simulink library "str"  (Simulink 8.2)
settings: Solver=ode45  SolverMode=SingleTasking  StartTime=0.0  StopTime=10.0  RelTol=1e-3
undefined symbols (not defined in the file or in its folder): ASTR_LFCTransGainIPTq_X_Nm, ASTR_LFCTransGainOPTq_X_Nm, ENUM_ADASLFCSTATUS_ACTIVE_NORMAL, ENUM_EPSMODEREQ_TORQUE, ENUM_LFCSTATE_SOFTEN, FALSE, KINP_SteerSpeedCalRate_s, KINP_SteerSpeedFltConst_s, KSTR_AngSvoErrGain_rat, KSTR_AngSvoFFVal_degps, KSTR_AngSvoIC_degps, KSTR_AngSvoIGain_rat, KSTR_AngSvoIMax_degps, KSTR_AngSvoIMin_degps, KSTR_AngSvoKGain_rat, KSTR_AngSvoPGain_rat, KSTR_ForceAngleServoOn_flg, KSTR_StrAngComdGain_rat, KSTR_StrAngGain_rat, KSTR_StrSpdGain_rat, KSTR_UseFakeStrAngReq_flg, MSTR_LFCTransGainIP_rat, MSTR_LFCTransGainOP_rat, TRUE
libraries: hcu_lib x6, simulink x3, inp x1
settings Model: Creator=13192  LastModifiedBy=13192

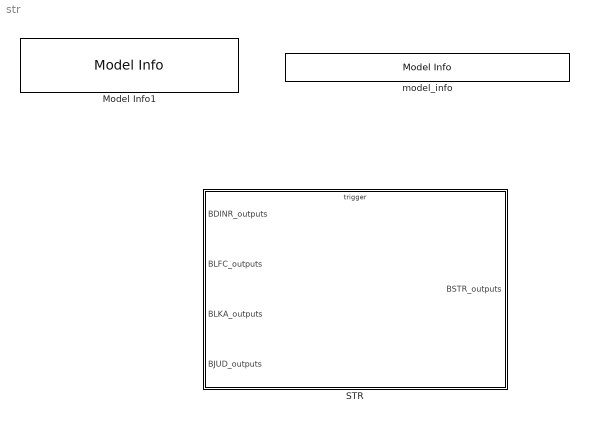
== system str ==
  Model Info1 : simulink/Model-Wide Utilities/Model Info  InitialBlockCM=None  BlockCM=None  Frame=on  DisplayStringWithTags=|  HorizontalTextAlignment=Left  LeftAlignmentValue=0.02  SourceBlockDiagram=str  TagMaxNumber=20
      | Model Version        : %<ModelVersion>
      | Creator                   : %<Creator>
      | Last Modified by    : %<LastModifiedBy>
  STR : Subsystem
      settings: RTWSystemCode=Nonreusable function  RTWFcnNameOpts=Use subsystem name  RTWFileNameOpts=Use subsystem name
  model_info : simulink/Model-Wide Utilities/Model Info  InitialBlockCM=None  BlockCM=None  Frame=on  DisplayStringWithTags=$Id: hcu_lib.mdl 289 2016-04-11 06:01:08Z chimotsai $  HorizontalTextAlignment=Center  LeftAlignmentValue=0.5  SourceBlockDiagram=str  TagMaxNumber=20

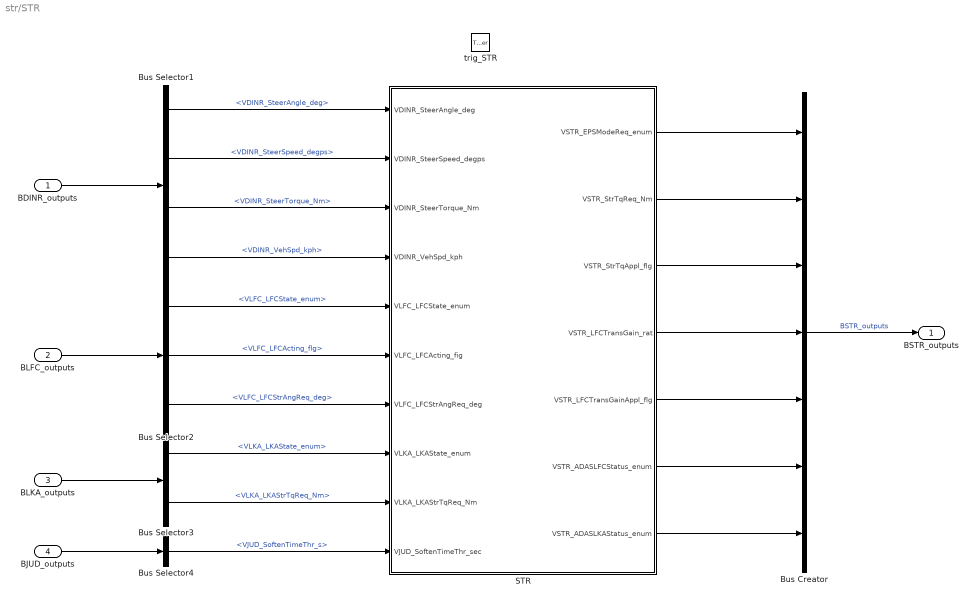
== system str/STR ==
  BDINR_outputs : Inport  OutDataTypeStr=Bus: BDINR_outputs
  BLFC_outputs : Inport  Port=2  OutDataTypeStr=Bus: BLFC_outputs
  BLKA_outputs : Inport  Port=3  OutDataTypeStr=Bus: BLKA_outputs
  BJUD_outputs : Inport  Port=4  OutDataTypeStr=Bus: BJUD_outputs
  trig_STR : TriggerPort  TriggerType=function-call
  Bus Creator : BusCreator  Inputs=7  OutDataTypeStr=Bus: BSTR_outputs
  Bus Selector1 : BusSelector  OutputSignals=VDINR_SteerAngle_deg,VDINR_SteerSpeed_degps,VDINR_SteerTorque_Nm,VDINR_VehSpd_kph
  Bus Selector2 : BusSelector  OutputSignals=VLFC_LFCState_enum,VLFC_LFCActing_flg,VLFC_LFCStrAngReq_deg
  Bus Selector3 : BusSelector  OutputSignals=VLKA_LKAState_enum,VLKA_LKAStrTqReq_Nm
  Bus Selector4 : BusSelector  OutputSignals=VJUD_SoftenTimeThr_s
  STR : Subsystem
  BSTR_outputs : Outport  OutDataTypeStr=Bus: BSTR_outputs
  wires:
  Bus Creator/1 -> BSTR_outputs/1  "BSTR_outputs"
  BDINR_outputs/1 -> Bus Selector1/1
  Bus Selector1/1 -> STR/1(VDINR_SteerAngle_deg)  "<VDINR_SteerAngle_deg>"
  Bus Selector1/2 -> STR/2(VDINR_SteerSpeed_degps)  "<VDINR_SteerSpeed_degps>"
  BLFC_outputs/1 -> Bus Selector2/1
  Bus Selector1/4 -> STR/4(VDINR_VehSpd_kph)  "<VDINR_VehSpd_kph>"
  Bus Selector2/1 -> STR/5(VLFC_LFCState_enum)  "<VLFC_LFCState_enum>"
  Bus Selector2/3 -> STR/7(VLFC_LFCStrAngReq_deg)  "<VLFC_LFCStrAngReq_deg>"
  BLKA_outputs/1 -> Bus Selector3/1
  Bus Selector3/1 -> STR/8(VLKA_LKAState_enum)  "<VLKA_LKAState_enum>"
  Bus Selector3/2 -> STR/9(VLKA_LKAStrTqReq_Nm)  "<VLKA_LKAStrTqReq_Nm>"
  Bus Selector1/3 -> STR/3(VDINR_SteerTorque_Nm)  "<VDINR_SteerTorque_Nm>"
  BJUD_outputs/1 -> Bus Selector4/1
  Bus Selector4/1 -> STR/10(VJUD_SoftenTimeThr_sec)  "<VJUD_SoftenTimeThr_s>"
  STR/1(VSTR_EPSModeReq_enum) -> Bus Creator/1
  STR/2(VSTR_StrTqReq_Nm) -> Bus Creator/2
  STR/3(VSTR_StrTqAppl_flg) -> Bus Creator/3
  STR/4(VSTR_LFCTransGain_rat) -> Bus Creator/4
  STR/5(VSTR_LFCTransGainAppl_flg) -> Bus Creator/5
  STR/6(VSTR_ADASLFCStatus_enum) -> Bus Creator/6
  STR/7(VSTR_ADASLKAStatus_enum) -> Bus Creator/7
  Bus Selector2/2 -> STR/6(VLFC_LFCActing_fig)  "<VLFC_LFCActing_flg>"

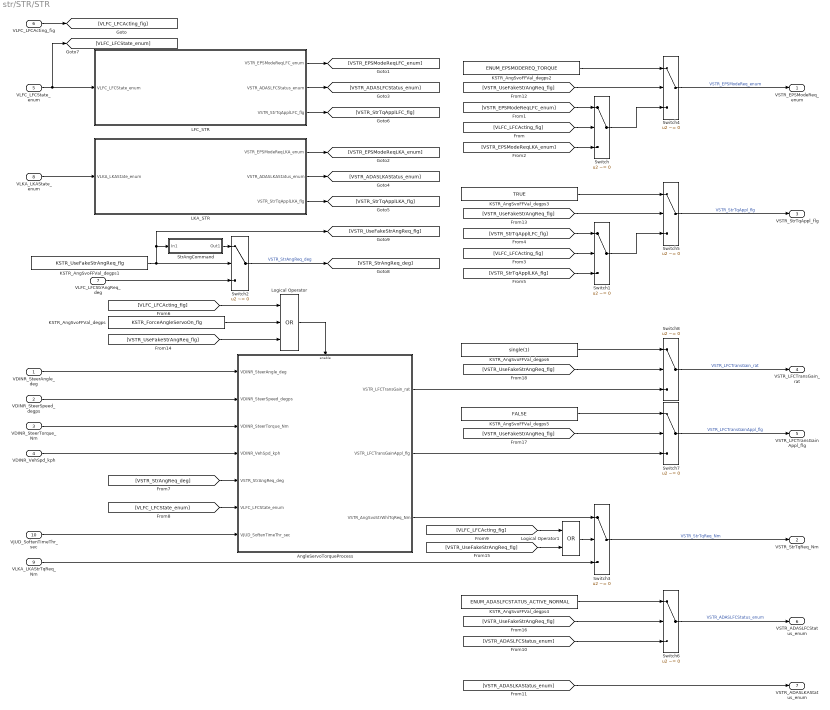
== system str/STR/STR ==
  VDINR_SteerAngle_deg : Inport
  VDINR_SteerSpeed_degps : Inport  Port=2
  VDINR_SteerTorque_Nm : Inport  Port=3
  VDINR_VehSpd_kph : Inport  Port=4
  VLFC_LFCState_enum : Inport  Port=5
  VLFC_LFCActing_fig : Inport  Port=6
  VLFC_LFCStrAngReq_deg : Inport  Port=7
  VLKA_LKAState_enum : Inport  Port=8
  VLKA_LKAStrTqReq_Nm : Inport  Port=9
  VJUD_SoftenTimeThr_sec : Inport  Port=10
  AngleServoTorqueProcess : Subsystem
  KSTR_AngSvoFFVal_degps : Constant  Value=KSTR_ForceAngleServoOn_flg
  KSTR_AngSvoFFVal_degps1 : Constant  Value=KSTR_UseFakeStrAngReq_flg
  KSTR_AngSvoFFVal_degps2 : Constant  Value=ENUM_EPSMODEREQ_TORQUE
  KSTR_AngSvoFFVal_degps3 : Constant  Value=TRUE
  KSTR_AngSvoFFVal_degps4 : Constant  Value=ENUM_ADASLFCSTATUS_ACTIVE_NORMAL
  KSTR_AngSvoFFVal_degps5 : Constant  Value=FALSE
  KSTR_AngSvoFFVal_degps6 : Constant  Value=single(1)
  LFC_STR : Stateflow chart  TreatAsAtomicUnit=on
  LKA_STR : Stateflow chart  TreatAsAtomicUnit=on
  Logical Operator : Logic  Operator=OR  Inputs=3  AllPortsSameDT=off  OutDataTypeStr=boolean
  Logical Operator1 : Logic  Operator=OR  AllPortsSameDT=off  OutDataTypeStr=boolean
  StrAngCommand : Subsystem
  Switch{,1..8} (9 alike) : Switch  Criteria=u2 ~= 0
  VSTR_EPSModeReq_enum : Outport
  VSTR_StrTqReq_Nm : Outport  Port=2
  VSTR_StrTqAppl_flg : Outport  Port=3
  VSTR_LFCTransGain_rat : Outport  Port=4
  VSTR_LFCTransGainAppl_flg : Outport  Port=5
  VSTR_ADASLFCStatus_enum : Outport  Port=6
  VSTR_ADASLKAStatus_enum : Outport  Port=7
  wires:
  VLKA_LKAState_enum/1 -> LKA_STR/1(VLKA_LKAState_enum)
  VLFC_LFCState_enum/1 -> [VLFC_LFCState_enum], LFC_STR/1(VLFC_LFCState_enum)
  VLFC_LFCActing_fig/1 -> [VLFC_LFCActing_fig]
  LFC_STR/1(VSTR_EPSModeReqLFC_enum) -> [VSTR_EPSModeReqLFC_enum]
  LKA_STR/1(VSTR_EPSModeReqLKA_enum) -> [VSTR_EPSModeReqLKA_enum]
  LFC_STR/2(VSTR_ADASLFCStatus_enum) -> [VSTR_ADASLFCStatus_enum]
  LKA_STR/2(VSTR_ADASLKAStatus_enum) -> [VSTR_ADASLKAStatus_enum]
  LKA_STR/3(VSTR_StrTqApplLKA_flg) -> [VSTR_StrTqApplLKA_flg]
  LFC_STR/3(VSTR_StrTqApplLFC_flg) -> [VSTR_StrTqApplLFC_flg]
  [VLFC_LFCActing_fig] -> Switch/2
  [VSTR_EPSModeReqLFC_enum] -> Switch/1
  [VSTR_EPSModeReqLKA_enum] -> Switch/3
  [VLFC_LFCActing_fig] -> Switch1/2
  [VSTR_StrTqApplLFC_flg] -> Switch1/1
  [VSTR_StrTqApplLKA_flg] -> Switch1/3
  Switch4/1 -> VSTR_EPSModeReq_enum/1  "VSTR_EPSModeReq_enum"
  Switch5/1 -> VSTR_StrTqAppl_flg/1  "VSTR_StrTqAppl_flg"
  Logical Operator/1 -> AngleServoTorqueProcess/Enable
  [VLFC_LFCActing_fig] -> Logical Operator/1
  KSTR_AngSvoFFVal_degps/1 -> Logical Operator/2
  VDINR_SteerAngle_deg/1 -> AngleServoTorqueProcess/1(VDINR_SteerAngle_deg)
  VDINR_SteerSpeed_degps/1 -> AngleServoTorqueProcess/2(VDINR_SteerSpeed_degps)
  VDINR_SteerTorque_Nm/1 -> AngleServoTorqueProcess/3(VDINR_SteerTorque_Nm)
  VDINR_VehSpd_kph/1 -> AngleServoTorqueProcess/4(VDINR_VehSpd_kph)
  KSTR_AngSvoFFVal_degps1/1 -> StrAngCommand/1(In1), [VSTR_UseFakeStrAngReq_flg], Switch2/2
  StrAngCommand/1(Out1) -> Switch2/1
  Switch2/1 -> [VSTR_StrAngReq_deg]  "VSTR_StrAngReq_deg"
  [VSTR_StrAngReq_deg] -> AngleServoTorqueProcess/5(VSTR_StrAngReq_deg)
  [VLFC_LFCState_enum] -> AngleServoTorqueProcess/6(VLFC_LFCState_enum)
  VJUD_SoftenTimeThr_sec/1 -> AngleServoTorqueProcess/7(VJUD_SoftenTimeThr_sec)
  VLKA_LKAStrTqReq_Nm/1 -> Switch3/3
  AngleServoTorqueProcess/3(VSTR_AngSvoStrWhlTqReq_Nm) -> Switch3/1
  Switch3/1 -> VSTR_StrTqReq_Nm/1  "VSTR_StrTqReq_Nm"
  AngleServoTorqueProcess/1(VSTR_LFCTransGain_rat) -> Switch8/3
  AngleServoTorqueProcess/2(VSTR_LFCTransGainAppl_flg) -> Switch7/3
  [VSTR_ADASLFCStatus_enum] -> Switch6/3
  [VSTR_ADASLKAStatus_enum] -> VSTR_ADASLKAStatus_enum/1
  [VSTR_UseFakeStrAngReq_flg] -> Switch4/2
  Switch/1 -> Switch4/3
  KSTR_AngSvoFFVal_degps2/1 -> Switch4/1
  [VSTR_UseFakeStrAngReq_flg] -> Switch5/2
  Switch1/1 -> Switch5/3
  KSTR_AngSvoFFVal_degps3/1 -> Switch5/1
  [VSTR_UseFakeStrAngReq_flg] -> Logical Operator/3
  Logical Operator1/1 -> Switch3/2
  [VLFC_LFCActing_fig] -> Logical Operator1/1
  [VSTR_UseFakeStrAngReq_flg] -> Logical Operator1/2
  [VSTR_UseFakeStrAngReq_flg] -> Switch6/2
  KSTR_AngSvoFFVal_degps4/1 -> Switch6/1
  Switch6/1 -> VSTR_ADASLFCStatus_enum/1  "VSTR_ADASLFCStatus_enum"
  [VSTR_UseFakeStrAngReq_flg] -> Switch7/2
  KSTR_AngSvoFFVal_degps5/1 -> Switch7/1
  Switch7/1 -> VSTR_LFCTransGainAppl_flg/1  "VSTR_LFCTransGainAppl_flg"
  [VSTR_UseFakeStrAngReq_flg] -> Switch8/2
  KSTR_AngSvoFFVal_degps6/1 -> Switch8/1
  Switch8/1 -> VSTR_LFCTransGain_rat/1  "VSTR_LFCTransGain_rat"
  VLFC_LFCStrAngReq_deg/1 -> Switch2/3

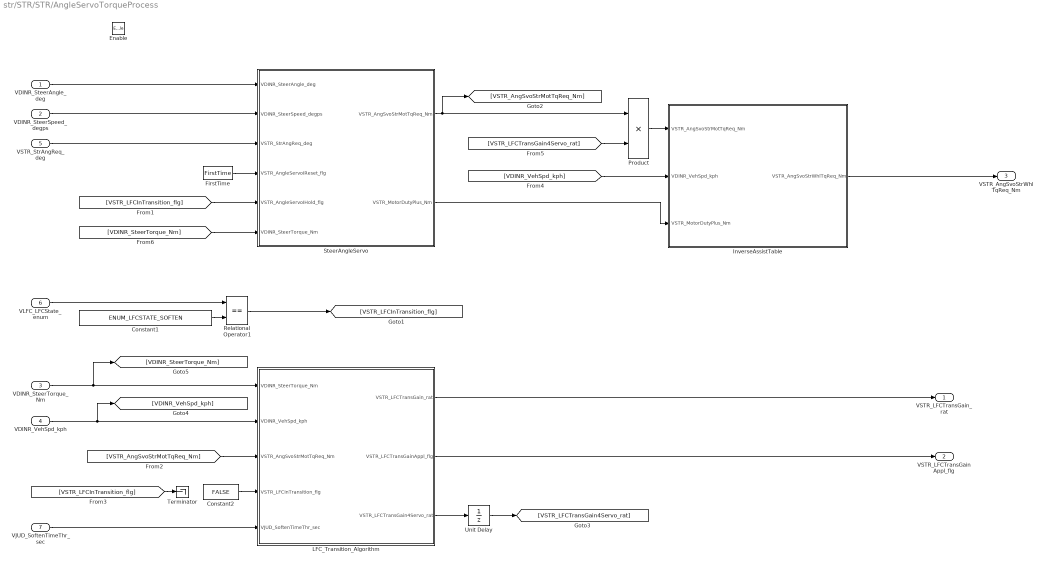
== system str/STR/STR/AngleServoTorqueProcess ==
  VDINR_SteerAngle_deg : Inport
  VDINR_SteerSpeed_degps : Inport  Port=2
  VDINR_SteerTorque_Nm : Inport  Port=3
  VDINR_VehSpd_kph : Inport  Port=4
  VSTR_StrAngReq_deg : Inport  Port=5
  VLFC_LFCState_enum : Inport  Port=6
  VJUD_SoftenTimeThr_sec : Inport  Port=7
  Enable : EnablePort  StatesWhenEnabling=reset
  Constant1 : Constant  Value=ENUM_LFCSTATE_SOFTEN
  Constant2 : Constant  Value=FALSE
  FirstTime : hcu_lib/FirstTime
  InverseAssistTable : Subsystem
  LFC_Transition_Algorithm : Subsystem
  Product : Product  Inputs=**
  Relational Operator1 : RelationalOperator  Operator===  OutDataTypeStr=boolean
  SteerAngleServo : Subsystem
  Terminator : Terminator
  Unit Delay : UnitDelay  InitialCondition=1  SampleTime=-1
  VSTR_LFCTransGain_rat : Outport  OutputWhenDisabled=reset  InitialOutput=[1]
  VSTR_LFCTransGainAppl_flg : Outport  Port=2  OutputWhenDisabled=reset  InitialOutput=[0]
  VSTR_AngSvoStrWhlTqReq_Nm : Outport  Port=3  OutputWhenDisabled=reset  InitialOutput=[0]
  wires:
  SteerAngleServo/1(VSTR_AngSvoStrMotTqReq_Nm) -> [VSTR_AngSvoStrMotTqReq_Nm], Product/1
  VDINR_SteerSpeed_degps/1 -> SteerAngleServo/2(VDINR_SteerSpeed_degps)
  VSTR_StrAngReq_deg/1 -> SteerAngleServo/3(VSTR_StrAngReq_deg)
  VDINR_SteerAngle_deg/1 -> SteerAngleServo/1(VDINR_SteerAngle_deg)
  InverseAssistTable/1(VSTR_AngSvoStrWhlTqReq_Nm) -> VSTR_AngSvoStrWhlTqReq_Nm/1
  FirstTime/1 -> SteerAngleServo/4(VSTR_AngleServoIReset_flg)
  VLFC_LFCState_enum/1 -> Relational Operator1/1
  Constant1/1 -> Relational Operator1/2
  [VSTR_LFCInTransition_flg] -> SteerAngleServo/5(VSTR_AngleServoIHold_flg)
  VDINR_VehSpd_kph/1 -> [VDINR_VehSpd_kph], LFC_Transition_Algorithm/2(VDINR_VehSpd_kph)
  VDINR_SteerTorque_Nm/1 -> [VDINR_SteerTorque_Nm], LFC_Transition_Algorithm/1(VDINR_SteerTorque_Nm)
  [VSTR_AngSvoStrMotTqReq_Nm] -> LFC_Transition_Algorithm/3(VSTR_AngSvoStrMotTqReq_Nm)
  [VSTR_LFCInTransition_flg] -> Terminator/1
  VJUD_SoftenTimeThr_sec/1 -> LFC_Transition_Algorithm/5(VJUD_SoftenTimeThr_sec)
  LFC_Transition_Algorithm/3(VSTR_LFCTransGain4Servo_rat) -> Unit Delay/1
  LFC_Transition_Algorithm/1(VSTR_LFCTransGain_rat) -> VSTR_LFCTransGain_rat/1
  LFC_Transition_Algorithm/2(VSTR_LFCTransGainAppl_flg) -> VSTR_LFCTransGainAppl_flg/1
  Unit Delay/1 -> [VSTR_LFCTransGain4Servo_rat]
  [VDINR_VehSpd_kph] -> InverseAssistTable/2(VDINR_VehSpd_kph)
  Product/1 -> InverseAssistTable/1(VSTR_AngSvoStrMotTqReq_Nm)
  [VSTR_LFCTransGain4Servo_rat] -> Product/2
  Constant2/1 -> LFC_Transition_Algorithm/4(VSTR_LFCInTransition_flg)
  SteerAngleServo/2(VSTR_MotorDutyPlus_Nm) -> InverseAssistTable/3(VSTR_MotorDutyPlus_Nm)
  Relational Operator1/1 -> [VSTR_LFCInTransition_flg]
  [VDINR_SteerTorque_Nm] -> SteerAngleServo/6(VDINR_SteerTorque_Nm)

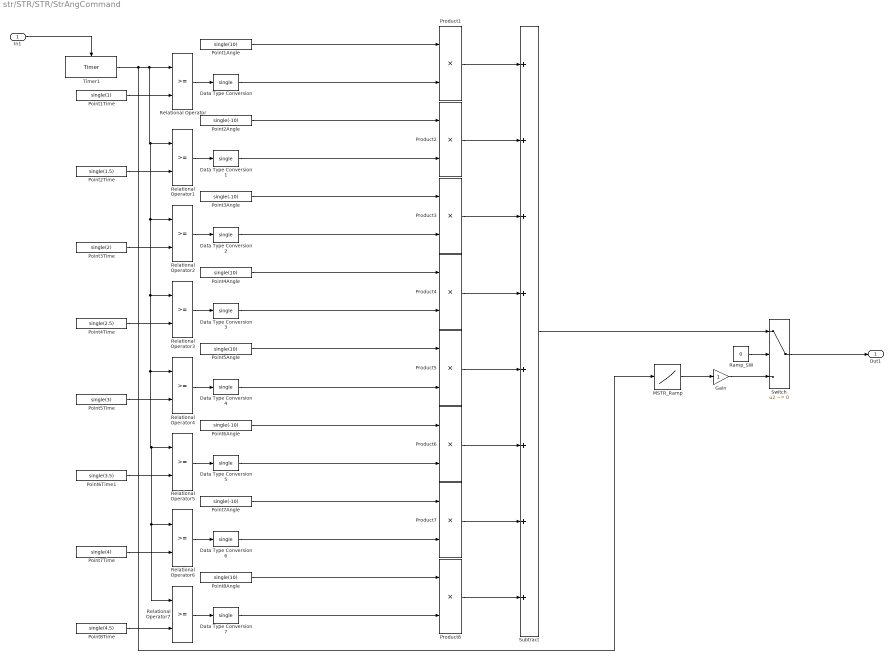
== system str/STR/STR/StrAngCommand ==
  In1 : Inport
  Data Type Conversion{,1..7} (8 alike) : DataTypeConversion  OutDataTypeStr=single
  Gain : Gain
  MSTR_Ramp : Lookup  InputValues=[0.5 1 1.1 3]  Table=[0 0 1 1]  LookUpMeth=Interpolation-Use End Values
      settings: AttributesFormatString="Input=\"%<InputValues>\"\\nOutput=\"%<Table>\""
  Point1Angle : Constant  Value=single(10)
  Point1Time : Constant  Value=single(1)
  Point2Angle : Constant  Value=single(-10)
  Point2Time : Constant  Value=single(1.5)
  Point3Angle : Constant  Value=single(-10)
  Point3Time : Constant  Value=single(2)
  Point4Angle : Constant  Value=single(10)
  Point4Time : Constant  Value=single(2.5)
  Point5Angle : Constant  Value=single(10)
  Point5Time : Constant  Value=single(3)
  Point6Angle : Constant  Value=single(-10)
  Point6Time1 : Constant  Value=single(3.5)
  Point7Angle : Constant  Value=single(-10)
  Point7Time : Constant  Value=single(4)
  Point8Angle : Constant  Value=single(10)
  Point8Time : Constant  Value=single(4.5)
  Product{1..8} (8 alike) : Product
  Ramp_SW : Constant  Value=0  OutDataTypeStr=boolean
  Relational Operator{,1..7} (8 alike) : RelationalOperator  OutDataTypeStr=boolean
  Subtract : Sum  Inputs=8
  Switch : Switch  Criteria=u2 ~= 0
  Timer1 : hcu_lib/Timer  SystemSampleTime=-1
  Out1 : Outport
  wires:
  In1/1 -> Timer1/Enable
  Point1Time/1 -> Relational Operator/2
  Relational Operator/1 -> Data Type Conversion/1
  Data Type Conversion/1 -> Product1/2
  Point1Angle/1 -> Product1/1
  Point2Time/1 -> Relational Operator1/2
  Data Type Conversion1/1 -> Product2/2
  Point2Angle/1 -> Product2/1
  Relational Operator1/1 -> Data Type Conversion1/1
  Point3Time/1 -> Relational Operator2/2
  Data Type Conversion2/1 -> Product3/2
  Relational Operator2/1 -> Data Type Conversion2/1
  Point3Angle/1 -> Product3/1
  Point4Time/1 -> Relational Operator3/2
  Data Type Conversion3/1 -> Product4/2
  Relational Operator3/1 -> Data Type Conversion3/1
  Point4Angle/1 -> Product4/1
  Point5Time/1 -> Relational Operator4/2
  Data Type Conversion4/1 -> Product5/2
  Relational Operator4/1 -> Data Type Conversion4/1
  Point5Angle/1 -> Product5/1
  Point6Time1/1 -> Relational Operator5/2
  Data Type Conversion5/1 -> Product6/2
  Relational Operator5/1 -> Data Type Conversion5/1
  Point6Angle/1 -> Product6/1
  Point7Time/1 -> Relational Operator6/2
  Data Type Conversion6/1 -> Product7/2
  Relational Operator6/1 -> Data Type Conversion6/1
  Point7Angle/1 -> Product7/1
  Timer1/1 -> MSTR_Ramp/1, Relational Operator7/1, Relational Operator6/1, Relational Operator5/1, Relational Operator4/1, Relational Operator3/1, Relational Operator2/1, Relational Operator1/1, Relational Operator/1
  Point8Time/1 -> Relational Operator7/2
  Data Type Conversion7/1 -> Product8/2
  Relational Operator7/1 -> Data Type Conversion7/1
  Point8Angle/1 -> Product8/1
  Product1/1 -> Subtract/1
  Product2/1 -> Subtract/2
  Product3/1 -> Subtract/3
  Product4/1 -> Subtract/4
  Product5/1 -> Subtract/5
  Product6/1 -> Subtract/6
  Product7/1 -> Subtract/7
  Product8/1 -> Subtract/8
  Switch/1 -> Out1/1
  MSTR_Ramp/1 -> Gain/1
  Subtract/1 -> Switch/1
  Gain/1 -> Switch/3
  Ramp_SW/1 -> Switch/2

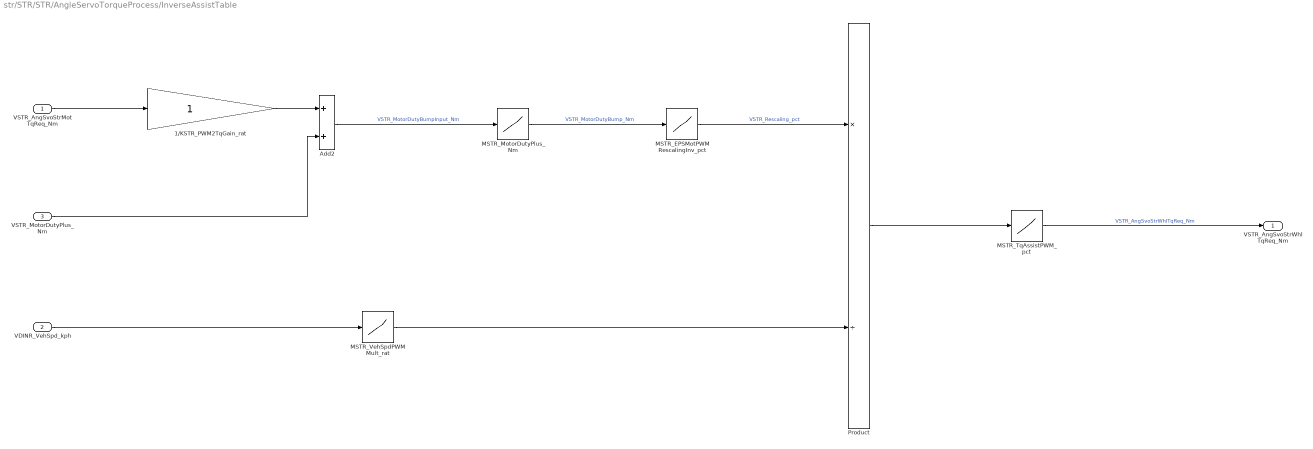
== system str/STR/STR/AngleServoTorqueProcess/InverseAssistTable ==
  VSTR_AngSvoStrMotTqReq_Nm : Inport
  VDINR_VehSpd_kph : Inport  Port=2
  VSTR_MotorDutyPlus_Nm : Inport  Port=3
  1/KSTR_PWM2TqGain_rat : Gain
  Add2 : Sum
  MSTR_EPSMotPWMRescalingInv_pct : Lookup  InputValues=[-250 -3 0 3 250]  Table=[-100 -3 0 3 100]  LookUpMeth=Interpolation-Use End Values
      settings: AttributesFormatString="Input=\"%<InputValues>\"\\nOutput=\"%<Table>\""
  MSTR_MotorDutyPlus_Nm : Lookup  InputValues=[-100 -50 -10 -5 -1 0 1 5 10 50 100]  Table=[-104 -54 -14 -9 -5 0 5 9 14 54 104]  LookUpMeth=Interpolation-Use End Values
      settings: AttributesFormatString="Input=\"%<InputValues>\"\\nOutput=\"%<Table>\""
  MSTR_TqAssistPWM_pct : Lookup  InputValues="[-100\t-95\t-90\t-85\t-80\t-75\t-70\t-65\t-60\t-55\t-50\t-45\t-40\t-35\t-30\t-25\t-20\t-15\t-10\t-5\t0\t5\t10\t15\t20\t25\t30\t35\t40\t45\t50\t55\t60\t65\t70\t75\t80\t85\t90\t95\t100]"  Table=[-10:0.5:10]  LookUpMeth=Interpolation-Use End Values
      settings: AttributesFormatString="Input=\"%<InputValues>\"\\nOutput=\"%<Table>\""
  MSTR_VehSpdPWMMult_rat : Lookup  InputValues=[-100 -80 -60 -40 -20 -10 0 10 20 40 60 80 100]  Table=[1 1 1 1 1 1 1 1 1 1 1 1 1]  LookUpMeth=Interpolation-Use End Values
      settings: AttributesFormatString="Input=\"%<InputValues>\"\\nOutput=\"%<Table>\""
  Product : Product  Inputs=*/
  VSTR_AngSvoStrWhlTqReq_Nm : Outport
  wires:
  VSTR_AngSvoStrMotTqReq_Nm/1 -> 1/KSTR_PWM2TqGain_rat/1
  1/KSTR_PWM2TqGain_rat/1 -> Add2/1
  VDINR_VehSpd_kph/1 -> MSTR_VehSpdPWMMult_rat/1
  MSTR_VehSpdPWMMult_rat/1 -> Product/2
  Product/1 -> MSTR_TqAssistPWM_pct/1
  MSTR_TqAssistPWM_pct/1 -> VSTR_AngSvoStrWhlTqReq_Nm/1  "VSTR_AngSvoStrWhlTqReq_Nm"
  MSTR_EPSMotPWMRescalingInv_pct/1 -> Product/1  "VSTR_Rescaling_pct"
  MSTR_MotorDutyPlus_Nm/1 -> MSTR_EPSMotPWMRescalingInv_pct/1  "VSTR_MotorDutyBump_Nm"
  Add2/1 -> MSTR_MotorDutyPlus_Nm/1  "VSTR_MotorDutyBumpInput_Nm"
  VSTR_MotorDutyPlus_Nm/1 -> Add2/2

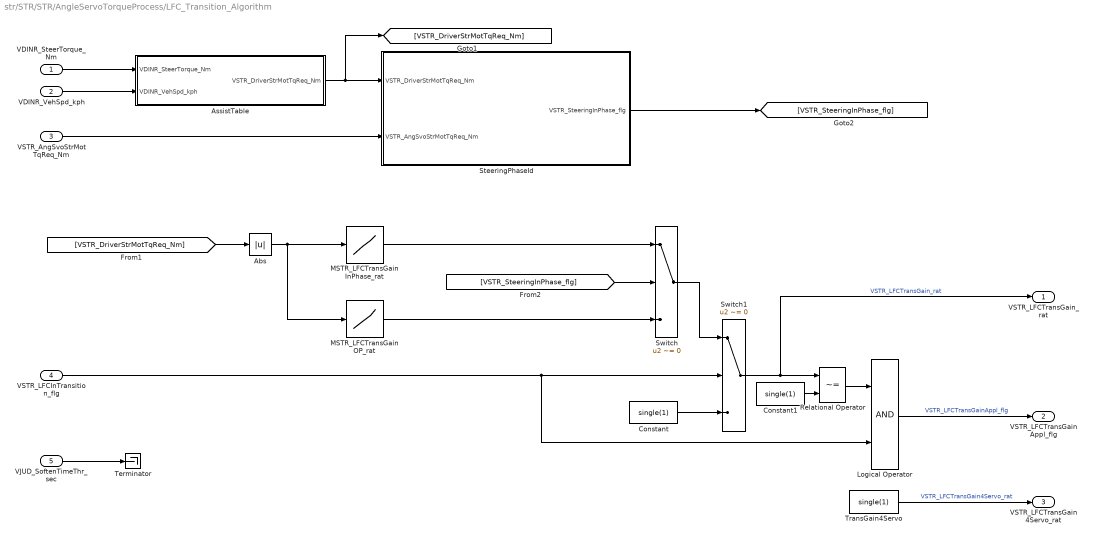
== system str/STR/STR/AngleServoTorqueProcess/LFC_Transition_Algorithm ==
  VDINR_SteerTorque_Nm : Inport
  VDINR_VehSpd_kph : Inport  Port=2
  VSTR_AngSvoStrMotTqReq_Nm : Inport  Port=3
  VSTR_LFCInTransition_flg : Inport  Port=4
  VJUD_SoftenTimeThr_sec : Inport  Port=5
  Abs : Abs
  AssistTable : Subsystem
  Constant : Constant  Value=single(1)
  Constant1 : Constant  Value=single(1)
  Logical Operator : Logic  AllPortsSameDT=off  OutDataTypeStr=boolean
  MSTR_LFCTransGainInPhase_rat : Lookup  InputValues=ASTR_LFCTransGainIPTq_X_Nm  Table=MSTR_LFCTransGainIP_rat  LookUpMeth=Interpolation-Use End Values
      settings: AttributesFormatString="Input=\"%<InputValues>\"\\nOutput=\"%<Table>\""
  MSTR_LFCTransGainOP_rat : Lookup  InputValues=ASTR_LFCTransGainOPTq_X_Nm  Table=MSTR_LFCTransGainOP_rat  LookUpMeth=Interpolation-Use End Values
      settings: AttributesFormatString="Input=\"%<InputValues>\"\\nOutput=\"%<Table>\""
  Relational Operator : RelationalOperator  Operator=~=  OutDataTypeStr=boolean
  SteeringPhaseId : Stateflow chart  TreatAsAtomicUnit=on
  Switch : Switch  Criteria=u2 ~= 0
  Switch1 : Switch  Criteria=u2 ~= 0
  Terminator : Terminator
  TransGain4Servo : Constant  Value=single(1)
  VSTR_LFCTransGain_rat : Outport  OutputWhenDisabled=reset  InitialOutput=[0]
  VSTR_LFCTransGainAppl_flg : Outport  Port=2  OutputWhenDisabled=reset  InitialOutput=[0]
  VSTR_LFCTransGain4Servo_rat : Outport  Port=3  OutputWhenDisabled=reset  InitialOutput=[0]
  wires:
  VSTR_AngSvoStrMotTqReq_Nm/1 -> SteeringPhaseId/2(VSTR_AngSvoStrMotTqReq_Nm)
  VDINR_SteerTorque_Nm/1 -> AssistTable/1(VDINR_SteerTorque_Nm)
  AssistTable/1(VSTR_DriverStrMotTqReq_Nm) -> [VSTR_DriverStrMotTqReq_Nm], SteeringPhaseId/1(VSTR_DriverStrMotTqReq_Nm)
  VDINR_VehSpd_kph/1 -> AssistTable/2(VDINR_VehSpd_kph)
  [VSTR_DriverStrMotTqReq_Nm] -> Abs/1
  Abs/1 -> MSTR_LFCTransGainInPhase_rat/1, MSTR_LFCTransGainOP_rat/1
  SteeringPhaseId/1(VSTR_SteeringInPhase_flg) -> [VSTR_SteeringInPhase_flg]
  [VSTR_SteeringInPhase_flg] -> Switch/2
  MSTR_LFCTransGainInPhase_rat/1 -> Switch/1
  MSTR_LFCTransGainOP_rat/1 -> Switch/3
  VSTR_LFCInTransition_flg/1 -> Logical Operator/2, Switch1/2
  Switch/1 -> Switch1/1
  Constant/1 -> Switch1/3
  Relational Operator/1 -> Logical Operator/1
  Switch1/1 -> VSTR_LFCTransGain_rat/1, Relational Operator/1  "VSTR_LFCTransGain_rat"
  Constant1/1 -> Relational Operator/2
  Logical Operator/1 -> VSTR_LFCTransGainAppl_flg/1  "VSTR_LFCTransGainAppl_flg"
  VJUD_SoftenTimeThr_sec/1 -> Terminator/1
  TransGain4Servo/1 -> VSTR_LFCTransGain4Servo_rat/1  "VSTR_LFCTransGain4Servo_rat"

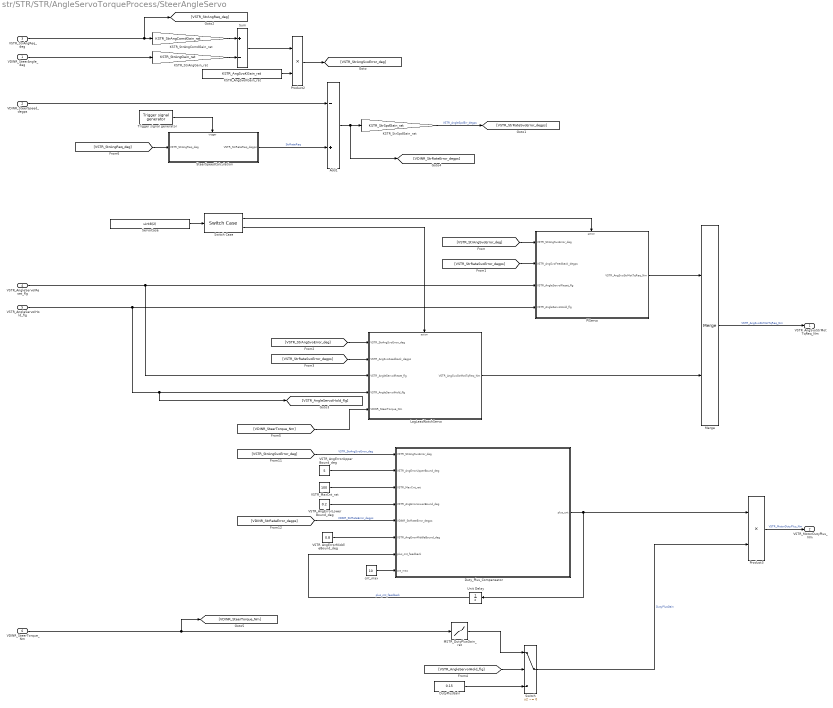
== system str/STR/STR/AngleServoTorqueProcess/SteerAngleServo ==
  VDINR_SteerAngle_deg : Inport
  VDINR_SteerSpeed_degps : Inport  Port=2
  VSTR_StrAngReq_deg : Inport  Port=3
  VSTR_AngleServoIReset_flg : Inport  Port=4
  VSTR_AngleServoIHold_flg : Inport  Port=5
  VDINR_SteerTorque_Nm : Inport  Port=6
  Add1 : Sum  Inputs=-+
  DutyPlusGain : Constant  Value=0.15  OutDataTypeStr=single
  Duty_Plus_Compensator : Stateflow chart  TreatAsAtomicUnit=on
  KSTR_AngSvoKGain_rat : Constant  Value=KSTR_AngSvoKGain_rat
  KSTR_StrAngComdGain_rat : Gain  Gain=KSTR_StrAngComdGain_rat
  KSTR_StrAngGain_rat : Gain  Gain=KSTR_StrAngGain_rat
  KSTR_StrSpdGain_rat : Gain  Gain=KSTR_StrSpdGain_rat
  LagLeadNotchServo : Subsystem
  MSTR_DutyPlusGain_rat : Lookup  InputValues=[1.25 1.5 1.75 2]  Table=[0 0 0 0]  LookUpMeth=Interpolation-Use End Values
      settings: AttributesFormatString="Input=\"%<InputValues>\"\\nOutput=\"%<Table>\""
  Merge : Merge
  PIServo : Subsystem
  Product2 : Product
  Product3 : Product
  ServoCase : Constant  Value=uint8(2)
  SteerSpeedCalculation : Subsystem
  Sum : Sum  Inputs=+-
  Switch : Switch  Criteria=u2 ~= 0
  Switch Case : SwitchCase  CaseConditions={1,2}  ShowDefaultCase=off
  Trigger signal generator : inp/INP/InputSignals/SignalProcess/Proc_SteerSpeedCal/Trigger signal generator
  Unit Delay : UnitDelay  SampleTime=-1
  VSTR_AngErrorLowerBound_deg : Constant  Value=0.2  OutDataTypeStr=single
  VSTR_AngErrorMiddleBound_deg : Constant  Value=0.8  OutDataTypeStr=single
  VSTR_AngErrorUpperBound_deg : Constant  Value=5  OutDataTypeStr=single
  VSTR_MaxCnt_rat : Constant  Value=100  OutDataTypeStr=single
  cnt_max : Constant  Value=10  OutDataTypeStr=single
  VSTR_AngSvoStrMotTqReq_Nm : Outport
  VSTR_MotorDutyPlus_Nm : Outport  Port=2
  wires:
  VSTR_StrAngReq_deg/1 -> [VSTR_StrAngReq_deg], KSTR_StrAngComdGain_rat/1
  KSTR_StrAngComdGain_rat/1 -> Sum/1
  KSTR_StrAngGain_rat/1 -> Sum/2
  Sum/1 -> Product2/1
  KSTR_AngSvoKGain_rat/1 -> Product2/2
  VDINR_SteerAngle_deg/1 -> KSTR_StrAngGain_rat/1
  KSTR_StrSpdGain_rat/1 -> [VSTR_StrRateSvoError_degps]  "VSTR_AngleSpdErr_degps"
  Product2/1 -> [VSTR_StrAngSvoError_deg]
  [VSTR_StrAngSvoError_deg] -> PIServo/1(VSTR_StrAngSvoError_deg)
  [VSTR_StrRateSvoError_degps] -> PIServo/2(VSTR_AngSvoFeedback_degps)
  VSTR_AngleServoIReset_flg/1 -> LagLeadNotchServo/3(VSTR_AngleServoIReset_flg), PIServo/3(VSTR_AngleServoIReset_flg)
  VSTR_AngleServoIHold_flg/1 -> LagLeadNotchServo/4(VSTR_AngleServoIHold_flg), [VSTR_AngleServoIHold_flg], PIServo/4(VSTR_AngleServoIHold_flg)
  PIServo/1(VSTR_AngSvoStrMotTqReq_Nm) -> Merge/1
  [VSTR_StrAngSvoError_deg] -> LagLeadNotchServo/1(VSTR_StrAngSvoError_deg)
  ServoCase/1 -> Switch Case/1
  Merge/1 -> VSTR_AngSvoStrMotTqReq_Nm/1  "VSTR_AngSvoStrMotTqReq_Nm"
  LagLeadNotchServo/1(VSTR_AngSvoStrMotTqReq_Nm) -> Merge/2
  Add1/1 -> KSTR_StrSpdGain_rat/1, [VDINR_StrRateError_degps]
  Trigger signal generator/1 -> SteerSpeedCalculation/Trigger
  [VSTR_StrAngReq_deg] -> SteerSpeedCalculation/1(VSTR_StrAngReq_deg)
  SteerSpeedCalculation/1(VSTR_StrRateReq_degps) -> Add1/2  "StrRateReq"
  [VSTR_StrRateSvoError_degps] -> LagLeadNotchServo/2(VSTR_AngSvoFeedback_degps)
  VDINR_SteerSpeed_degps/1 -> Add1/1
  [VSTR_StrAngSvoError_deg] -> Duty_Plus_Compensator/1(VSTR_StrAngSvoError_deg)  "VSTR_StrAngSvoError_deg"
  Duty_Plus_Compensator/1(plus_cnt) -> Unit Delay/1, Product3/1
  Product3/1 -> VSTR_MotorDutyPlus_Nm/1  "VSTR_MotorDutyPlus_Nm"
  VSTR_AngErrorUpperBound_deg/1 -> Duty_Plus_Compensator/2(VSTR_AngErrorUpperBound_deg)
  VSTR_MaxCnt_rat/1 -> Duty_Plus_Compensator/3(VSTR_MaxCnt_rat)
  VSTR_AngErrorLowerBound_deg/1 -> Duty_Plus_Compensator/4(VSTR_AngErrorLowerBound_deg)
  VSTR_AngErrorMiddleBound_deg/1 -> Duty_Plus_Compensator/6(VSTR_AngErrorMiddleBound_deg)
  [VDINR_StrRateError_degps] -> Duty_Plus_Compensator/5(VDINR_StrRateError_degps)  "VDINR_StrRateError_degps"
  Switch Case/1 -> PIServo/Action
  Switch Case/2 -> LagLeadNotchServo/Action
  Unit Delay/1 -> Duty_Plus_Compensator/7(plus_cnt_feedback)  "plus_cnt_feedback"
  cnt_max/1 -> Duty_Plus_Compensator/8(cnt_max)
  Switch/1 -> Product3/2  "DutyPlusGain"
  DutyPlusGain/1 -> Switch/3
  [VSTR_AngleServoIHold_flg] -> Switch/2
  MSTR_DutyPlusGain_rat/1 -> Switch/1
  VDINR_SteerTorque_Nm/1 -> [VDINR_SteerTorque_Nm], MSTR_DutyPlusGain_rat/1
  [VDINR_SteerTorque_Nm] -> LagLeadNotchServo/5(VDINR_SteerTorque_Nm)

== system str/STR/STR/AngleServoTorqueProcess/LFC_Transition_Algorithm/AssistTable ==
  VDINR_SteerTorque_Nm : Inport
  VDINR_VehSpd_kph : Inport  Port=2
  KSTR_PWM2TqGain_rat : Gain
  MSTR_MotorPWMRescaling_pct : Lookup  InputValues=[-100 -3 0 3 100]  Table=[-250 -3 0 3 250]  LookUpMeth=Interpolation-Use End Values
      settings: AttributesFormatString="Input=\"%<InputValues>\"\\nOutput=\"%<Table>\""
  MSTR_TqPWM_pct : Lookup  InputValues=[-10:0.5:10]  Table="[-100\t-95\t-90\t-85\t-80\t-75\t-70\t-65\t-60\t-55\t-50\t-45\t-40\t-35\t-30\t-25\t-20\t-15\t-10\t-5\t0\t5\t10\t15\t20\t25\t30\t35\t40\t45\t50\t55\t60\t65\t70\t75\t80\t85\t90\t95\t100]"  LookUpMeth=Interpolation-Use End Values
      settings: AttributesFormatString="Input=\"%<InputValues>\"\\nOutput=\"%<Table>\""
  MSTR_VehSpdPWMMult_rat : Lookup  InputValues=[-100 -80 -60 -40 -20 -10 0 10 20 40 60 80 100]  Table=[1 1 1 1 1 1 1 1 1 1 1 1 1]  LookUpMeth=Interpolation-Use End Values
      settings: AttributesFormatString="Input=\"%<InputValues>\"\\nOutput=\"%<Table>\""
  Product : Product  Inputs=**
  VSTR_DriverStrMotTqReq_Nm : Outport
  wires:
  VDINR_VehSpd_kph/1 -> MSTR_VehSpdPWMMult_rat/1
  MSTR_VehSpdPWMMult_rat/1 -> Product/2
  KSTR_PWM2TqGain_rat/1 -> VSTR_DriverStrMotTqReq_Nm/1  "VSTR_DriverStrMotTqReq_Nm"
  VDINR_SteerTorque_Nm/1 -> MSTR_TqPWM_pct/1
  MSTR_TqPWM_pct/1 -> Product/1
  MSTR_MotorPWMRescaling_pct/1 -> KSTR_PWM2TqGain_rat/1
  Product/1 -> MSTR_MotorPWMRescaling_pct/1

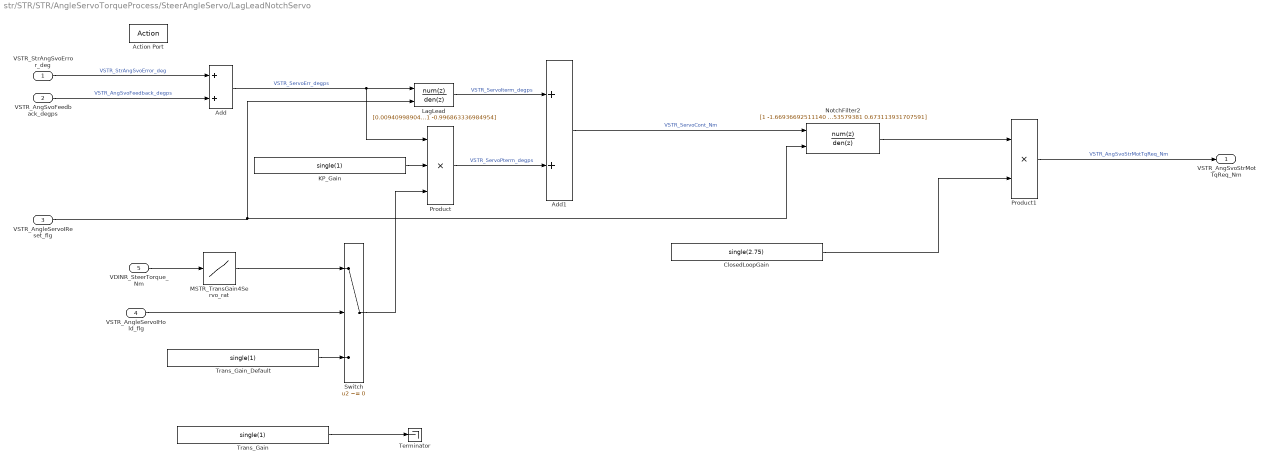
== system str/STR/STR/AngleServoTorqueProcess/SteerAngleServo/LagLeadNotchServo ==
  VSTR_StrAngSvoError_deg : Inport
  VSTR_AngSvoFeedback_degps : Inport  Port=2
  VSTR_AngleServoIReset_flg : Inport  Port=3
  VSTR_AngleServoIHold_flg : Inport  Port=4
  VDINR_SteerTorque_Nm : Inport  Port=5
  Action Port : ActionPort  ActionType=case
  Add : Sum
  Add1 : Sum
  ClosedLoopGain : Constant  Value=single(2.75)
  KP_Gain : Constant  Value=single(1)
  LagLead : DiscreteTransferFcn  Numerator=[0.00940998904513760]  Denominator=[1 -0.996863336984954]  ExternalReset=Rising
      settings: InputPortMap=u0,r7
  MSTR_TransGain4Servo_rat : Lookup  InputValues=[1.25 1.5 1.75 2 2.25]  Table=[1 0.9 0.8 0.7 0.6]  LookUpMeth=Interpolation-Use End Values
      settings: AttributesFormatString="Input=\"%<InputValues>\"\\nOutput=\"%<Table>\""
  NotchFilter2 : DiscreteTransferFcn  Numerator=[1 -1.66936692511140 0.709143321025187]  Denominator=[1 -1.63333753579381 0.673113931707591]  ExternalReset=Rising
      settings: InputPortMap=u0,r7
  Product : Product  Inputs=3
  Product1 : Product
  Switch : Switch  Criteria=u2 ~= 0
  Terminator : Terminator
  Trans_Gain : Constant  Value=single(1)
  Trans_Gain_Default : Constant  Value=single(1)
  VSTR_AngSvoStrMotTqReq_Nm : Outport  OutputWhenDisabled=reset  InitialOutput=[0]
  wires:
  Product1/1 -> VSTR_AngSvoStrMotTqReq_Nm/1  "VSTR_AngSvoStrMotTqReq_Nm"
  VSTR_StrAngSvoError_deg/1 -> Add/1  "VSTR_StrAngSvoError_deg"
  VSTR_AngSvoFeedback_degps/1 -> Add/2  "VSTR_AngSvoFeedback_degps"
  Add/1 -> LagLead/1, Product/1  "VSTR_ServoErr_degps"
  LagLead/1 -> Add1/1  "VSTR_ServoIterm_degps"
  Product/1 -> Add1/2  "VSTR_ServoPterm_degps"
  Add1/1 -> NotchFilter2/1  "VSTR_ServoCont_Nm"
  ClosedLoopGain/1 -> Product1/2
  VSTR_AngleServoIReset_flg/1 -> LagLead/2, NotchFilter2/2
  VSTR_AngleServoIHold_flg/1 -> Switch/2
  NotchFilter2/1 -> Product1/1
  KP_Gain/1 -> Product/2
  Switch/1 -> Product/3
  Trans_Gain_Default/1 -> Switch/3
  VDINR_SteerTorque_Nm/1 -> MSTR_TransGain4Servo_rat/1
  MSTR_TransGain4Servo_rat/1 -> Switch/1
  Trans_Gain/1 -> Terminator/1

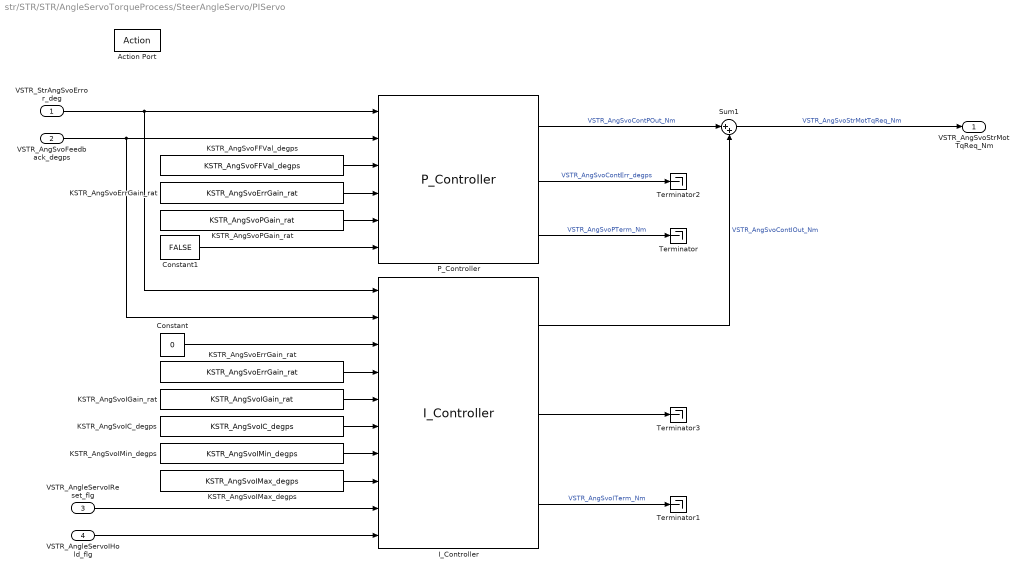
== system str/STR/STR/AngleServoTorqueProcess/SteerAngleServo/PIServo ==
  VSTR_StrAngSvoError_deg : Inport
  VSTR_AngSvoFeedback_degps : Inport  Port=2
  VSTR_AngleServoIReset_flg : Inport  Port=3
  VSTR_AngleServoIHold_flg : Inport  Port=4
  Action Port : ActionPort  ActionType=case
  Constant : Constant  Value=0  OutDataTypeStr=single
  Constant1 : Constant  Value=FALSE  OutDataTypeStr=single
  I_Controller : hcu_lib/I_Controller  SystemSampleTime=-1
  KSTR_AngSvoErrGain_rat : Constant  Value=KSTR_AngSvoErrGain_rat
  "KSTR_AngSvoErrGain_rat " : Constant  Value=KSTR_AngSvoErrGain_rat
  KSTR_AngSvoFFVal_degps : Constant  Value=KSTR_AngSvoFFVal_degps
  KSTR_AngSvoIC_degps : Constant  Value=KSTR_AngSvoIC_degps
  KSTR_AngSvoIGain_rat : Constant  Value=KSTR_AngSvoIGain_rat
  KSTR_AngSvoIMax_degps : Constant  Value=KSTR_AngSvoIMax_degps
  KSTR_AngSvoIMin_degps : Constant  Value=KSTR_AngSvoIMin_degps
  KSTR_AngSvoPGain_rat : Constant  Value=KSTR_AngSvoPGain_rat
  P_Controller : hcu_lib/P_Controller  SystemSampleTime=-1
  Sum1 : Sum  Inputs=|++
  Terminator{,1..3} (4 alike) : Terminator
  VSTR_AngSvoStrMotTqReq_Nm : Outport  OutputWhenDisabled=reset  InitialOutput=[0]
  wires:
  KSTR_AngSvoIMin_degps/1 -> I_Controller/7
  KSTR_AngSvoIC_degps/1 -> I_Controller/6
  KSTR_AngSvoPGain_rat/1 -> P_Controller/5
  Constant1/1 -> P_Controller/6
  KSTR_AngSvoIGain_rat/1 -> I_Controller/5
  I_Controller/1 -> Sum1/2  "VSTR_AngSvoContIOut_Nm"
  Constant/1 -> I_Controller/3
  I_Controller/2 -> Terminator3/1
  P_Controller/1 -> Sum1/1  "VSTR_AngSvoContPOut_Nm"
  "KSTR_AngSvoErrGain_rat "/1 -> I_Controller/4
  KSTR_AngSvoErrGain_rat/1 -> P_Controller/4
  KSTR_AngSvoFFVal_degps/1 -> P_Controller/3
  VSTR_AngSvoFeedback_degps/1 -> I_Controller/2, P_Controller/2
  VSTR_StrAngSvoError_deg/1 -> I_Controller/1, P_Controller/1
  VSTR_AngleServoIHold_flg/1 -> I_Controller/10
  Sum1/1 -> VSTR_AngSvoStrMotTqReq_Nm/1  "VSTR_AngSvoStrMotTqReq_Nm"
  VSTR_AngleServoIReset_flg/1 -> I_Controller/9
  P_Controller/2 -> Terminator2/1  "VSTR_AngSvoContErr_degps"
  I_Controller/3 -> Terminator1/1  "VSTR_AngSvoITerm_Nm"
  KSTR_AngSvoIMax_degps/1 -> I_Controller/8
  P_Controller/3 -> Terminator/1  "VSTR_AngSvoPTerm_Nm"

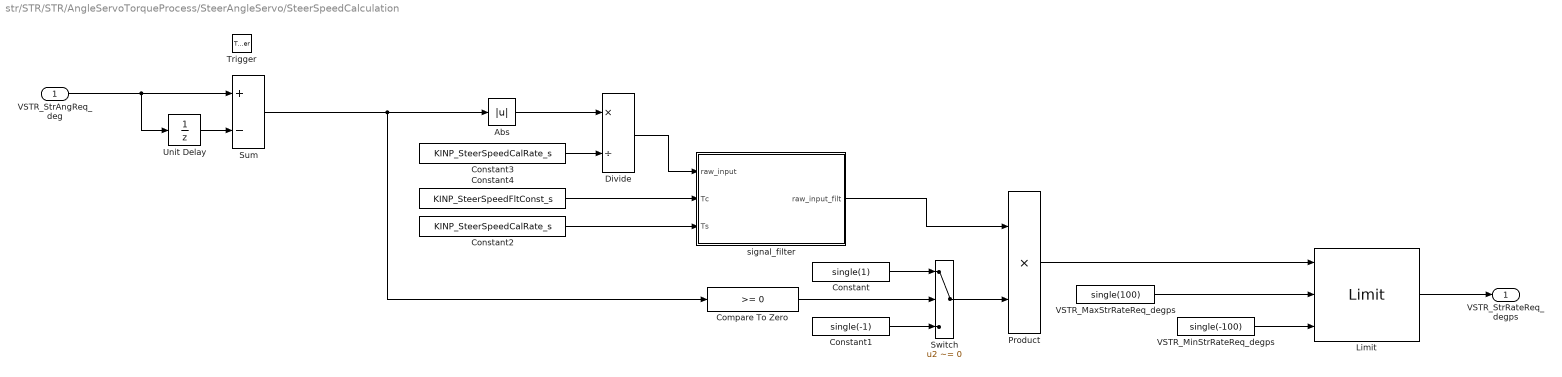
== system str/STR/STR/AngleServoTorqueProcess/SteerAngleServo/SteerSpeedCalculation ==
  VSTR_StrAngReq_deg : Inport
  Trigger : TriggerPort
  Abs : Abs
  Compare To Zero : simulink/Logic and Bit Operations/Compare To Zero  relop=>=  OutDataTypeStr=boolean
  Constant : Constant  Value=single(1)
  Constant1 : Constant  Value=single(-1)
  Constant2 : Constant  Value=KINP_SteerSpeedCalRate_s
  Constant3 : Constant  Value=KINP_SteerSpeedCalRate_s
  Constant4 : Constant  Value=KINP_SteerSpeedFltConst_s
  Divide : Product  Inputs=*/
  Limit : hcu_lib/Limit  SystemSampleTime=-1
  Product : Product
  Sum : Sum  Inputs=+-
  Switch : Switch  Criteria=u2 ~= 0
  Unit Delay : UnitDelay  SampleTime=-1
  VSTR_MaxStrRateReq_degps : Constant  Value=single(100)
  VSTR_MinStrRateReq_degps : Constant  Value=single(-100)
  signal_filter : Subsystem
  VSTR_StrRateReq_degps : Outport
  wires:
  signal_filter/1(raw_input_filt) -> Product/1
  Switch/1 -> Product/2
  Constant1/1 -> Switch/3
  Constant/1 -> Switch/1
  Compare To Zero/1 -> Switch/2
  Constant3/1 -> Divide/2
  Abs/1 -> Divide/1
  Sum/1 -> Compare To Zero/1, Abs/1
  Unit Delay/1 -> Sum/2
  Constant2/1 -> signal_filter/3(Ts)
  Constant4/1 -> signal_filter/2(Tc)
  Divide/1 -> signal_filter/1(raw_input)
  VSTR_StrAngReq_deg/1 -> Sum/1, Unit Delay/1
  Product/1 -> Limit/1
  Limit/1 -> VSTR_StrRateReq_degps/1
  VSTR_MaxStrRateReq_degps/1 -> Limit/2
  VSTR_MinStrRateReq_degps/1 -> Limit/3

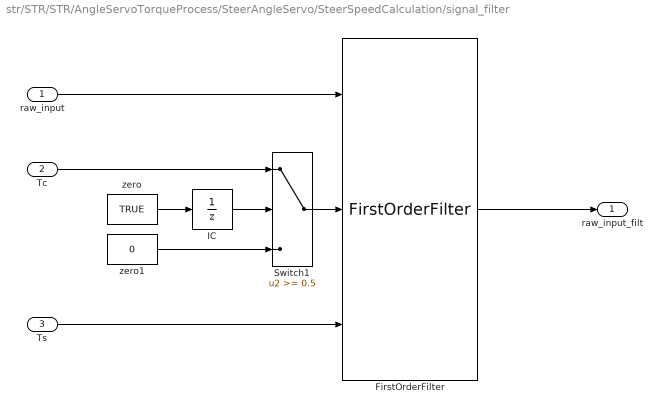
== system str/STR/STR/AngleServoTorqueProcess/SteerAngleServo/SteerSpeedCalculation/signal_filter ==
  raw_input : Inport
  Tc : Inport  Port=2
  Ts : Inport  Port=3
  FirstOrderFilter : hcu_lib/FirstOrderFilter  SystemSampleTime=-1
  IC : UnitDelay  Tag=struct('comment',struct('text','','placement',1),'logdata',struct('maxnumvals',inf,'plotchannels',[],'stepsize',0,'downsampling',1,'loggingmode',3,'channels',1),'output',struct('width',1,'name','$S_$B','unit','','type','Int16','offset',0,'max',NaN,'min',NaN,'freeze',1,'lsb',1,'arb',0,'class','default','address','','description','','autoscalingmode',1,'lowerheadroom',1,'upperheadroom',1,'headroomunit','bit','checkmin',0,'checkmax',0,'show',0,'initial','2'),'state',0,'dt','-1','date',731455.586925799)  SampleTime=-1
  Switch1 : Switch  Tag=struct('comment',struct('text','','placement',1),'logdata',struct('maxnumvals',inf,'plotchannels',[],'stepsize',0,'downsampling',1,'loggingmode',3,'channels',1),'output',struct('width',1,'name','$S_$B','unit','','type','Int32Bin15','offset',0,'max',65535,'min',-65536,'freeze',1,'lsb',2^-15,'arb',0,'class','default','address','','description','','autoscalingmode',1,'lowerheadroom',1,'upperheadroom',1,'headroomunit','bit','checkmin',0,'checkmax',0,'show',0),'threshold',struct('width',1,'name','$S_$B_threshold','unit','','type','Int16','offset',0,'max',NaN,'min',NaN,'freeze',1,'lsb',1,'arb',0,'class','default','address','','description','','value','1','scalar',0),'date',731455.58657044)  Threshold=0.5  InputSameDT=on
  zero : Constant  Tag=struct('comment',struct('text','','placement',1),'output',struct('width',1,'name','$S_$B','unit','','type','Int16','offset',0,'max',NaN,'min',NaN,'freeze',1,'lsb',1,'arb',0,'class','default','address','','description','','value','0','tolerance',1,'show',0),'date',731455.58675544)  Value=TRUE
  zero1 : Constant  Tag=struct('comment',struct('text','','placement',1),'output',struct('width',1,'name','$S_$B','unit','','type','Int16','offset',0,'max',NaN,'min',NaN,'freeze',1,'lsb',1,'arb',0,'class','default','address','','description','','value','0','tolerance',1,'show',0),'date',731455.58675544)  Value=0  OutDataTypeStr=single
  raw_input_filt : Outport
  wires:
  zero/1 -> IC/1
  raw_input/1 -> FirstOrderFilter/1
  Tc/1 -> Switch1/1
  Ts/1 -> FirstOrderFilter/3
  IC/1 -> Switch1/2
  FirstOrderFilter/1 -> raw_input_filt/1
  Switch1/1 -> FirstOrderFilter/2
  zero1/1 -> Switch1/3

== stateflow chart STR/STR/AngleServoTorqueProcess/LFC_Transition_Algorithm/SteeringPhaseId ==
  (default) -> (junction 8)
  (junction 8) -> (junction 9) [order 1] : [VSTR_DriverStrMotTqReq_Nm >= 0 && ...
      | VSTR_AngSvoStrMotTqReq_Nm >= 0]
  (junction 8) -> (junction 10) [order 2]
  (junction 9) -> (junction 14) : {VSTR_SteeringInPhase_flg=TRUE;}
  (junction 10) -> (junction 11) [order 1] : [VSTR_DriverStrMotTqReq_Nm < 0 && ...
      | VSTR_AngSvoStrMotTqReq_Nm < 0]
  (junction 10) -> (junction 12) [order 2] : {VSTR_SteeringInPhase_flg=FALSE;}
  (junction 11) -> (junction 13) : {VSTR_SteeringInPhase_flg=TRUE;}
  (junction 13) -> (junction 12)
  (junction 14) -> (junction 13)
  data: VSTR_DriverStrMotTqReq_Nm input double; VSTR_AngSvoStrMotTqReq_Nm input double; VSTR_SteeringInPhase_flg output double; TRUE parameter double; FALSE parameter double

== stateflow chart STR/STR/AngleServoTorqueProcess/SteerAngleServo/Duty_Plus_Compensator ==
  (default) -> (junction 35)
  (junction 35) -> (junction 36) [order 1] : [abs(VSTR_StrAngSvoError_deg) < VSTR_AngErrorUpperBound_deg]
  (junction 35) -> (junction 37) [order 2]
  (junction 36) -> (junction 41)
  (junction 37) -> (junction 38) [order 1] : [plus_cnt == 0 ]
  (junction 37) -> (junction 39) [order 2]
  (junction 38) -> (junction 84) : {plus_cnt = 0;}
  (junction 39) -> (junction 40) [order 1] : [plus_cnt > 0 && plus_cnt_feedback > 0]
  (junction 39) -> (junction 51) [order 2]
  (junction 40) -> (junction 45) : {plus_cnt = plus_cnt -cnt_max;}
  (junction 41) -> (junction 42) [order 1] : [VSTR_StrAngSvoError_deg > VSTR_AngErrorLowerBound_deg && VDINR_StrRateError_degps >= 0]
  (junction 41) -> (junction 43) [order 2]
  (junction 42) -> (junction 47)
  (junction 43) -> (junction 44) [order 1] : [VSTR_StrAngSvoError_deg < -VSTR_AngErrorLowerBound_deg && VDINR_StrRateError_degps <= 0]
  (junction 43) -> (junction 85) [order 2]
  (junction 44) -> (junction 49)
  (junction 45) -> (junction 46) [order 1] : [plus_cnt < 0]
  (junction 47) -> (junction 48) [order 1] : [plus_cnt >= 0]
  (junction 45) -> (junction 82) [order 2]
  (junction 46) -> (junction 83) : {plus_cnt = 0;}
  (junction 47) -> (junction 53) [order 2]
  (junction 48) -> (junction 55)
  (junction 49) -> (junction 50) [order 1] : [plus_cnt <= 0]
  (junction 49) -> (junction 57) [order 2]
  (junction 50) -> (junction 59)
  (junction 51) -> (junction 52) [order 1] : [plus_cnt < 0 && plus_cnt_feedback < 0]
  (junction 51) -> (junction 79) [order 2]
  (junction 52) -> (junction 61) : {plus_cnt = plus_cnt + cnt_max;}
  (junction 53) -> (junction 54) [order 1] : [VSTR_StrAngSvoError_deg > VSTR_AngErrorMiddleBound_deg]
  (junction 55) -> (junction 56) [order 1] : [VSTR_StrAngSvoError_deg > VSTR_AngErrorMiddleBound_deg]
  (junction 53) -> (junction 63) [order 2] : {plus_cnt = plus_cnt +2;}
  (junction 54) -> (junction 64) : {plus_cnt = plus_cnt +4;}
  (junction 57) -> (junction 58) [order 1] : [VSTR_StrAngSvoError_deg < -VSTR_AngErrorMiddleBound_deg]
  (junction 59) -> (junction 60) [order 1] : [VSTR_StrAngSvoError_deg < -VSTR_AngErrorMiddleBound_deg]
  (junction 55) -> (junction 69) [order 2] : {plus_cnt = plus_cnt +1;}
  (junction 56) -> (junction 70) : {plus_cnt = plus_cnt +2;}
  (junction 57) -> (junction 65) [order 2] : {plus_cnt = plus_cnt -2;}
  (junction 58) -> (junction 66) : {plus_cnt = plus_cnt -4;}
  (junction 59) -> (junction 67) [order 2] : {plus_cnt = plus_cnt -1;}
  (junction 60) -> (junction 68) : {plus_cnt = plus_cnt -2;}
  (junction 61) -> (junction 62) [order 1] : [plus_cnt>0]
  (junction 61) -> (junction 80) [order 2]
  (junction 62) -> (junction 81) : {plus_cnt=0;}
  (junction 64) -> (junction 63)
  (junction 63) -> (junction 71)
  (junction 66) -> (junction 65)
  (junction 68) -> (junction 67)
  (junction 70) -> (junction 69)
  (junction 65) -> (junction 75)
  (junction 67) -> (junction 77)
  (junction 69) -> (junction 73)
  (junction 71) -> (junction 72) [order 1] : [plus_cnt >= VSTR_MaxCnt_rat]
  (junction 73) -> (junction 74) [order 1] : [plus_cnt >= VSTR_MaxCnt_rat]
  (junction 71) -> (junction 90) [order 2]
  (junction 72) -> (junction 91) : {plus_cnt = VSTR_MaxCnt_rat;}
  (junction 73) -> (junction 92) [order 2]
  (junction 74) -> (junction 93) : {plus_cnt = VSTR_MaxCnt_rat;}
  (junction 75) -> (junction 76) [order 1] : [plus_cnt <= -VSTR_MaxCnt_rat]
  (junction 77) -> (junction 78) [order 1] : [plus_cnt <= -VSTR_MaxCnt_rat]
  (junction 75) -> (junction 86) [order 2]
  (junction 76) -> (junction 87) : {plus_cnt = -VSTR_MaxCnt_rat;}
  (junction 77) -> (junction 88) [order 2]
  (junction 78) -> (junction 89) : {plus_cnt = -VSTR_MaxCnt_rat;}
  (junction 80) -> (junction 79)
  (junction 81) -> (junction 80)
  (junction 82) -> (junction 81)
  (junction 83) -> (junction 82)
  (junction 84) -> (junction 83)
  (junction 85) -> (junction 84)
  (junction 86) -> (junction 85)
  (junction 87) -> (junction 86)
  (junction 88) -> (junction 87)
  (junction 89) -> (junction 88)
  (junction 90) -> (junction 89)
  (junction 91) -> (junction 90)
  (junction 92) -> (junction 91)
  (junction 93) -> (junction 92)
  data: VSTR_StrAngSvoError_deg input single; plus_cnt output single; VSTR_AngErrorUpperBound_deg input single; VSTR_MaxCnt_rat input single; VSTR_AngErrorLowerBound_deg input single; VDINR_StrRateError_degps input single; VSTR_AngErrorMiddleBound_deg input single; plus_cnt_feedback input single; cnt_max input single

== stateflow chart STR/STR/LFC_STR ==
  (default) -> (junction 194)
  (junction 194) -> (junction 195) [order 1] : [VLFC_LFCState_enum==ENUM_LFCSTATE_DISABLED]
  (junction 194) -> (junction 196) [order 2]
  (junction 195) -> (junction 218) : {VSTR_EPSModeReqLFC_enum=ENUM_EPSMODEREQ_INTERNAL; ...
      | VSTR_ADASLFCStatus_enum=ENUM_ADASLFCSTATUS_OFF; ...
      | VSTR_StrTqApplLFC_flg=FALSE;}
  (junction 196) -> (junction 197) [order 1] : [VLFC_LFCState_enum==ENUM_LFCSTATE_OFF]
  (junction 196) -> (junction 198) [order 2]
  (junction 197) -> (junction 217) : {VSTR_EPSModeReqLFC_enum=ENUM_EPSMODEREQ_INTERNAL; ...
      | VSTR_ADASLFCStatus_enum=ENUM_ADASLFCSTATUS_OFF; ...
      | VSTR_StrTqApplLFC_flg=FALSE;}
  (junction 198) -> (junction 199) [order 1] : [VLFC_LFCState_enum==ENUM_LFCSTATE_STANDBY]
  (junction 198) -> (junction 200) [order 2]
  (junction 199) -> (junction 216) : {VSTR_EPSModeReqLFC_enum=ENUM_EPSMODEREQ_INTERNAL; ...
      | VSTR_ADASLFCStatus_enum=ENUM_ADASLFCSTATUS_STANDBY; ...
      | VSTR_StrTqApplLFC_flg=FALSE;}
  (junction 200) -> (junction 201) [order 1] : [VLFC_LFCState_enum==ENUM_LFCSTATE_AUTOSTEERING]
  (junction 200) -> (junction 202) [order 2]
  (junction 201) -> (junction 215) : {VSTR_EPSModeReqLFC_enum=ENUM_EPSMODEREQ_TORQUE; ...
      | VSTR_ADASLFCStatus_enum=ENUM_ADASLFCSTATUS_ACTIVE_NORMAL; ...
      | VSTR_StrTqApplLFC_flg=TRUE;}
  (junction 202) -> (junction 203) [order 1] : [VLFC_LFCState_enum==ENUM_LFCSTATE_DEGRADED]
  (junction 202) -> (junction 204) [order 2]
  (junction 203) -> (junction 214) : {VSTR_EPSModeReqLFC_enum=ENUM_EPSMODEREQ_TORQUE; ...
      | VSTR_ADASLFCStatus_enum=ENUM_ADASLFCSTATUS_ACTIVE_NORMAL; ...
      | VSTR_StrTqApplLFC_flg=TRUE;}
  (junction 204) -> (junction 205) [order 1] : [VLFC_LFCState_enum==ENUM_LFCSTATE_SOFTEN]
  (junction 204) -> (junction 206) [order 2]
  (junction 205) -> (junction 213) : {VSTR_EPSModeReqLFC_enum=ENUM_EPSMODEREQ_TORQUE; ...
      | VSTR_ADASLFCStatus_enum=ENUM_ADASLFCSTATUS_ACTIVE_TRANSITION; ...
      | VSTR_StrTqApplLFC_flg=TRUE;}
  (junction 206) -> (junction 207) [order 1] : [VLFC_LFCState_enum==ENUM_LFCSTATE_ADASFAILURE]
  (junction 206) -> (junction 208) [order 2]
  (junction 207) -> (junction 212) : {VSTR_EPSModeReqLFC_enum=ENUM_EPSMODEREQ_INTERNAL; ...
      | VSTR_ADASLFCStatus_enum=ENUM_ADASLFCSTATUS_NOTAVAIL_TEMP; ...
      | VSTR_StrTqApplLFC_flg=FALSE;}
  (junction 208) -> (junction 209) [order 1] : [VLFC_LFCState_enum==ENUM_LFCSTATE_EPSRECOVERYPENDING]
  (junction 208) -> (junction 210) [order 2] : {VSTR_EPSModeReqLFC_enum=ENUM_EPSMODEREQ_INTERNAL; ...
      | VSTR_ADASLFCStatus_enum=ENUM_ADASLFCSTATUS_OFF; ...
      | VSTR_StrTqApplLFC_flg=FALSE;}
  (junction 209) -> (junction 211) : {VSTR_EPSModeReqLFC_enum=ENUM_EPSMODEREQ_INTERNAL; ...
      | VSTR_ADASLFCStatus_enum=ENUM_ADASLFCSTATUS_OFF; ...
      | VSTR_StrTqApplLFC_flg=FALSE;}
  (junction 211) -> (junction 210)
  (junction 212) -> (junction 211)
  (junction 213) -> (junction 212)
  (junction 214) -> (junction 213)
  (junction 215) -> (junction 214)
  (junction 216) -> (junction 215)
  (junction 217) -> (junction 216)
  (junction 218) -> (junction 217)
  data: VLFC_LFCState_enum input double; VSTR_EPSModeReqLFC_enum output double; VSTR_ADASLFCStatus_enum output double; VSTR_StrTqApplLFC_flg output double; ENUM_LFCSTATE_DISABLED parameter double; ENUM_LFCSTATE_OFF parameter double; ENUM_LFCSTATE_STANDBY parameter double; ENUM_LFCSTATE_AUTOSTEERING parameter double; ENUM_LFCSTATE_DEGRADED parameter double; ENUM_LFCSTATE_SOFTEN parameter double; ENUM_LFCSTATE_ADASFAILURE parameter double; ENUM_LFCSTATE_EPSRECOVERYPENDING parameter double; ENUM_EPSMODEREQ_INTERNAL parameter double; ENUM_EPSMODEREQ_TORQUE parameter double; ENUM_ADASLFCSTATUS_OFF parameter double; ENUM_ADASLFCSTATUS_STANDBY parameter double; ENUM_ADASLFCSTATUS_ACTIVE_NORMAL parameter double; ENUM_ADASLFCSTATUS_ACTIVE_TRANSITION parameter double; ENUM_ADASLFCSTATUS_NOTAVAIL_TEMP parameter double; TRUE parameter double; FALSE parameter double

== stateflow chart STR/STR/LKA_STR ==
  (default) -> (junction 273)
  (junction 273) -> (junction 274) [order 1] : [VLKA_LKAState_enum==ENUM_LKASTATE_DISABLED]
  (junction 273) -> (junction 275) [order 2]
  (junction 274) -> (junction 294) : {VSTR_EPSModeReqLKA_enum=ENUM_EPSMODEREQ_INTERNAL; ...
      | VSTR_ADASLKAStatus_enum=ENUM_ADASLKASTATUS_OFF; ...
      | VSTR_StrTqApplLKA_flg=FALSE;}
  (junction 275) -> (junction 276) [order 1] : [VLKA_LKAState_enum==ENUM_LKASTATE_OFF]
  (junction 275) -> (junction 277) [order 2]
  (junction 276) -> (junction 293) : {VSTR_EPSModeReqLKA_enum=ENUM_EPSMODEREQ_INTERNAL; ...
      | VSTR_ADASLKAStatus_enum=ENUM_ADASLKASTATUS_OFF; ...
      | VSTR_StrTqApplLKA_flg=FALSE;}
  (junction 277) -> (junction 278) [order 1] : [VLKA_LKAState_enum==ENUM_LKASTATE_STANDBY]
  (junction 277) -> (junction 279) [order 2]
  (junction 278) -> (junction 292) : {VSTR_EPSModeReqLKA_enum=ENUM_EPSMODEREQ_INTERNAL; ...
      | VSTR_ADASLKAStatus_enum=ENUM_ADASLKASTATUS_STANDBY; ...
      | VSTR_StrTqApplLKA_flg=FALSE;}
  (junction 279) -> (junction 280) [order 1] : [VLKA_LKAState_enum==ENUM_LKASTATE_OPERATIONAL]
  (junction 279) -> (junction 281) [order 2]
  (junction 280) -> (junction 291) : {VSTR_EPSModeReqLKA_enum=ENUM_EPSMODEREQ_INTERNAL; ...
      | VSTR_ADASLKAStatus_enum=ENUM_ADASLKASTATUS_STANDBY; ...
      | VSTR_StrTqApplLKA_flg=FALSE;}
  (junction 281) -> (junction 282) [order 1] : [VLKA_LKAState_enum==ENUM_LKASTATE_LEFTASSISTING || ...
      | VLKA_LKAState_enum==ENUM_LKASTATE_RIGHTASSISTING]
  (junction 281) -> (junction 283) [order 2]
  (junction 282) -> (junction 290) : {VSTR_EPSModeReqLKA_enum=ENUM_EPSMODEREQ_INTERNAL; ...
      | VSTR_ADASLKAStatus_enum=ENUM_ADASLKASTATUS_ACTIVE; ...
      | VSTR_StrTqApplLKA_flg=TRUE;}
  (junction 283) -> (junction 284) [order 1] : [VLKA_LKAState_enum==ENUM_LKASTATE_ADASFAILURE]
  (junction 283) -> (junction 285) [order 2]
  (junction 284) -> (junction 289) : {VSTR_EPSModeReqLKA_enum=ENUM_EPSMODEREQ_INTERNAL; ...
      | VSTR_ADASLKAStatus_enum=ENUM_ADASLKASTATUS_NOTAVAIL_TEMP; ...
      | VSTR_StrTqApplLKA_flg=FALSE;}
  (junction 285) -> (junction 286) [order 1] : [VLKA_LKAState_enum==ENUM_LKASTATE_EPSRECOVERYPENDING]
  (junction 285) -> (junction 287) [order 2] : {VSTR_EPSModeReqLKA_enum=ENUM_EPSMODEREQ_INTERNAL; ...
      | VSTR_ADASLKAStatus_enum=ENUM_ADASLKASTATUS_OFF; ...
      | VSTR_StrTqApplLKA_flg=FALSE;}
  (junction 286) -> (junction 288) : {VSTR_EPSModeReqLKA_enum=ENUM_EPSMODEREQ_INTERNAL; ...
      | VSTR_ADASLKAStatus_enum=ENUM_ADASLKASTATUS_OFF; ...
      | VSTR_StrTqApplLKA_flg=FALSE;}
  (junction 288) -> (junction 287)
  (junction 289) -> (junction 288)
  (junction 290) -> (junction 289)
  (junction 291) -> (junction 290)
  (junction 292) -> (junction 291)
  (junction 293) -> (junction 292)
  (junction 294) -> (junction 293)
  data: VLKA_LKAState_enum input double; VSTR_EPSModeReqLKA_enum output double; VSTR_ADASLKAStatus_enum output double; VSTR_StrTqApplLKA_flg output double; TRUE parameter double; FALSE parameter double; ENUM_LKASTATE_DISABLED parameter double; ENUM_LKASTATE_OFF parameter double; ENUM_LKASTATE_STANDBY parameter double; ENUM_LKASTATE_OPERATIONAL parameter double; ENUM_LKASTATE_RIGHTASSISTING parameter double; ENUM_LKASTATE_ADASFAILURE parameter double; ENUM_LKASTATE_EPSRECOVERYPENDING parameter double; ENUM_EPSMODEREQ_INTERNAL parameter double; ENUM_ADASLKASTATUS_OFF parameter double; ENUM_ADASLKASTATUS_STANDBY parameter double; ENUM_ADASLKASTATUS_ACTIVE parameter double; ENUM_ADASLKASTATUS_NOTAVAIL_TEMP parameter double; ENUM_LKASTATE_LEFTASSISTING parameter double
